simulink model "DifferentialRobotV1"  (R2020b)
settings: Solver=FixedStepAuto  StartTime=0.0  StopTime=1  FixedStep=0.01  RelTol=1e-3
values from neighbouring files (symbols this model uses):
  l = 100    [RobotInput.mat]
settings Model: Creator=AA  LastModifiedBy=AA

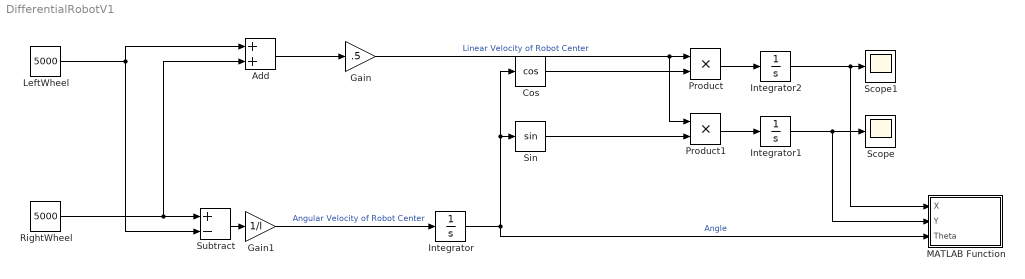
== system DifferentialRobotV1 ==
  Add : Sum
  Cos : Trigonometry  Operator=cos
  Gain : Gain  Gain=.5
  Gain1 : Gain  Gain=1/l
  Integrator : Integrator
  Integrator1 : Integrator  InitialCondition=1000
  Integrator2 : Integrator  InitialCondition=1000
  LeftWheel : Constant  Value=5000
  MATLAB Function : MATLAB Function  TreatAsAtomicUnit=on
  Product : Product  RndMeth=Zero
  Product1 : Product  RndMeth=Zero
  RightWheel : Constant  Value=5000
  Scope : Scope
  Scope1 : Scope
  Sin : Trigonometry
  Subtract : Sum  Inputs=+-
  wires:
  LeftWheel/1 -> Subtract/2, Add/1
  RightWheel/1 -> Subtract/1, Add/2
  Add/1 -> Gain/1
  Subtract/1 -> Gain1/1
  Gain1/1 -> Integrator/1  "Angular Velocity of Robot Center"
  Integrator/1 -> Sin/1, Cos/1, MATLAB Function/3(Theta)  "Angle"
  Gain/1 -> Product/1, Product1/1  "Linear Velocity of Robot Center"
  Cos/1 -> Product/2
  Sin/1 -> Product1/2
  Product/1 -> Integrator2/1
  Product1/1 -> Integrator1/1
  Integrator1/1 -> MATLAB Function/2(Y), Scope/1
  Integrator2/1 -> MATLAB Function/1(X), Scope1/1

== matlab function DifferentialRobotV1/MATLAB Function ==
  data: X input; Y input; Theta input
function fcn(X,Y,Theta)
%% Robot Construction
th = 0:pi/50:2*pi;
RobotR = 100;
xunit = RobotR * cos(th) + X;
yunit = RobotR * sin(th) + Y;
% Robot Direction
RobotVector = 200;
VectorX = linspace(X,RobotVector*cos(Theta) + X);
VectorY = linspace(Y,RobotVector*sin(Theta) + Y);

%% middle Circle
[xcircle, ycircle] = circle(5200,3700,500);
%% Edge Coordinates
OuterEdgeX =[linspace(0,0) linspace(0,10400) linspace(10400,10400) linspace(10400,0)];
OuterEdgeY =[linspace(0,7400) linspace(7400,7400) linspace(7400,0) linspace(0,0)];   
InnerEdgeX = [linspace(400,400) linspace(400,10000) linspace(10000,10000) linspace(10000,400)];
InnerEdgeY = [linspace(400,7000) linspace(7000,7000) linspace(7000,400) linspace(400,400)]; 
PlayEdgeX = [linspace(700,700) linspace(700,9700) linspace(9700,9700) linspace(9700,700)];               
PlayEdgeY = [linspace(700,6700) linspace(6700,6700) linspace(6700,700) linspace(700,700)];
%% Horizontal Line of playground
x1 = linspace(700,9700);
y1 = linspace(3700,3700);
%% Vertical Line of playground
y2 = linspace(700,6700);
x2 = linspace(5200,5200);
%% Defence Area edges
defx0 =linspace(700,1700); defx1 = linspace(1700,1700);  defx2= linspace(1700,700); % 
defx00 =linspace(8700,9700); defx11 = linspace(8700,8700);  defx22= linspace(8700,9700);
defy0 =linspace(2700,2700);defy1 = linspace(2700,4700);  defy2= linspace(4700,4700);
Defx =[ defx0 defx1 defx2]; Defy = [defy0 defy1 defy2];
Defxx = [defx00 defx11 defx22]; Defyy = Defy;
%% Goal
Goalx0 =linspace(700,500); Goalx1 = linspace(500,500);  Goalx2= linspace(500,700);
Goaly0 =linspace(3200,3200); Goaly1 = linspace(3200,4200);  Goaly2= linspace(4200,4200);
Goalx =[ Goalx0 Goalx1 Goalx2]; Goaly = [Goaly0 Goaly1 Goaly2];
Goalx00 =linspace(9700,9900); Goalx11 = linspace(9900,9900);  Goalx22= linspace(9900,9700);
Goalxx =[ Goalx00 Goalx11 Goalx22]; Goalyy = Goaly;
%% Plot
plot(x1,y1,'g',x2,y2,'g',Defx,Defy,'g',Defxx,Defyy,'g',Goalx,Goaly,'r',Goalxx,Goalyy,'r',xunit,yunit,VectorX,VectorY,OuterEdgeX,OuterEdgeY,'g',InnerEdgeX,InnerEdgeY,'g',PlayEdgeX,PlayEdgeY,'g',xcircle,ycircle,'g')
xlim([0 10400])
ylim([0 7400])
